simulink model "ODE_Hand_Model_v08_IPC_v02"  (Simulink 7.5)
settings: Solver=FixedStepDiscrete  StartTime=0.0  StopTime=inf  FixedStep=0.0315/(4*12)  RelTol=1e-3
values from neighbouring files (symbols this model uses):
  f_step = 0.7    [Set_Parameters.m]
  force_step = 20    [Set_Parameters.m]
  K_Conn = eye(4)*k_conn    [Set_Parameters.m]
  K_D = 30    [Set_Parameters.m]
  K_Or = eye(3)*k_Or    [Set_Parameters.m]
  K_Ot = eye(3)*k_Ot    [Set_Parameters.m]
  K_P = 350    [Set_Parameters.m]
  ksi = 2.0    (= 2)    [Set_Parameters.m]
  Kx = diag([diag(K_Ot)' diag(K_Or)' diag(K_Conn)'])    [Set_Parameters.m]
  l_des = [l1_des; l2_des; l3_des; l4_des]    [Set_Parameters.m]
  Mo = diag([sphere_mass*ones(1,3) (2/5)*sphere_mass*sphere_radius^2*ones(1,3)])    [Set_Parameters.m]
  qd_initial_touch = [0 0.3655   -0.5897   -0.5897     0       -0.3333   +0.5942   +0.5942         0       -0.298   --0.5226   --0.5226           0       -0.3333   +0.5942   +0.5942]    [Set_Parameters.m]
  R_O_Desired = R_O(x_i(qd_initial_touch))    [Set_Parameters.m]
  t_f_start = 2.5    [Set_Parameters.m]
  torque_step = 60    [Set_Parameters.m]
  x_O_desired = (1/4)*sum(x_i(qd_initial_touch))    [Set_Parameters.m]
undefined symbols (not defined in the file or in its folder): sigbuilder_block, skew
libraries: dspmtrx3 x29, simulink x4, dspinverses x1
settings Model: Creator=nihil  LastModifiedBy=konstantinos  SimulationMode=external
settings HardwareCC: ProdIntDivRoundTo=Zero  ProdEndianess=LittleEndian  ProdHWDeviceType=Generic->32-bit x86 compatible
settings RTWCC: SystemTargetFile=rtwin.tlc  TemplateMakefile=rtwin.tmf  Description=Real-Time Windows Target  ProcessScript=rtwin_make_rtw_hook  RTWCompilerOptimization=On
settings CodeAppCC: MaxIdLength=95
settings RTWinTargetCC: TargetLibSuffix=_rtwin.lib  TargetPreCompLibLocation=C:\Program Files (x86)\MATLAB\R2010a\toolbox\rtw\targets\rtwin\lib  TargetFunctionLibrary=ANSI_C  ERTCodeCoverageTool=None  PortableWordSizes=off

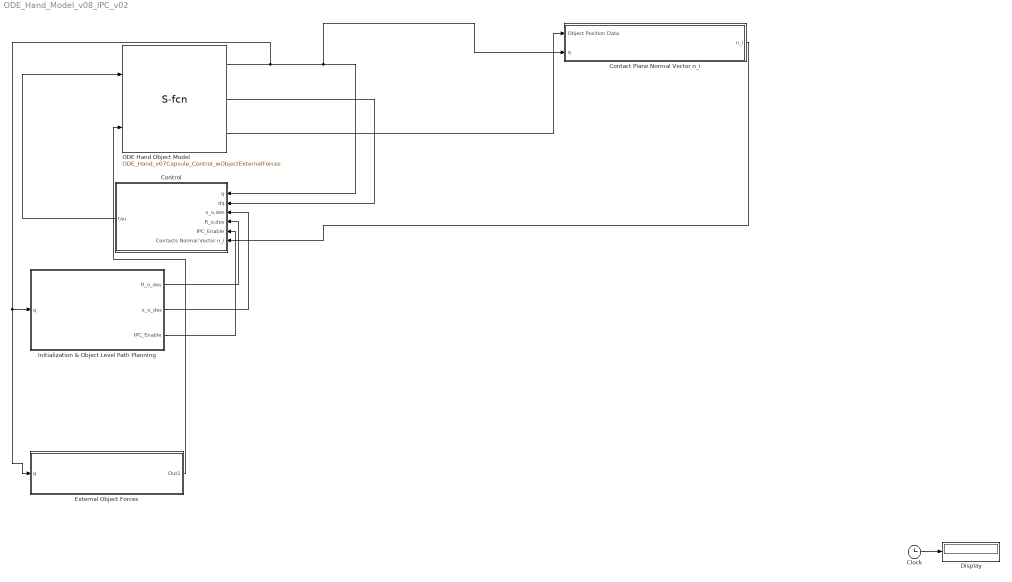
== system ODE_Hand_Model_v08_IPC_v02 ==
  Clock : Clock
      settings: Decimation=10
  Contact Plane Normal Vector n_i : Subsystem
  Control : Subsystem
  Display : Display
  External Object Forces : Subsystem
  Initialization & Object Level Path Planning : Subsystem
  ODE Hand Object Model : S-Function  FunctionName=ODE_Hand_v07Capsule_Control_wObjectExternalForces  EnableBusSupport=off
  wires:
  Clock/1 -> Display/1
  Control/1(tau) -> ODE Hand Object Model/1
  ODE Hand Object Model/1 -> Contact Plane Normal Vector n_i/2(q), Control/1(q), External Object Forces/1(q), Initialization & Object Level Path Planning/1(q)
  ODE Hand Object Model/2 -> Control/2(dq)
  Initialization & Object Level Path Planning/2(x_o_des) -> Control/3(x_o,des)
  Initialization & Object Level Path Planning/1(R_o_des) -> Control/4(R_o,des)
  Initialization & Object Level Path Planning/3(IPC_Enable) -> Control/5(IPC_Enable)
  External Object Forces/1(Out1) -> ODE Hand Object Model/2
  Contact Plane Normal Vector n_i/1(n_i) -> Control/6(Contacts Normal Vector n_i)
  ODE Hand Object Model/3 -> Contact Plane Normal Vector n_i/1(Object Position Data)

== system ODE_Hand_Model_v08_IPC_v02/Contact Plane Normal Vector n_i ==
  Object Position Data : Inport  OutDataType=fixdt(1, 16)  OutScaling=2^0
  q : Inport  Port=2  OutDataType=fixdt(1, 16)  OutScaling=2^0
  Cylindrical Object : Subsystem
  Manual Switch : simulink/Signal Routing/Manual Switch  SystemSampleTime=-1  sw=0  action=0  varsize=off
  Sphere : Subsystem
  x_i : MATLABFcn  MATLABFcn=x_i  Output1D=off
  n_i : Outport  OutDataType=fixdt(1, 16)  OutScaling=2^0
  wires:
  Object Position Data/1 -> Sphere/1(In1), Cylindrical Object/1(Position_Orientation)
  Sphere/1(Out1) -> Manual Switch/1
  Cylindrical Object/1(Out1) -> Manual Switch/2
  Manual Switch/1 -> n_i/1
  x_i/1 -> Cylindrical Object/2(x_i), Sphere/2(In2)
  q/1 -> x_i/1

== system ODE_Hand_Model_v08_IPC_v02/Control ==
  q : Inport  OutDataType=fixdt(1, 16)  OutScaling=2^0
  dq : Inport  Port=2  OutDataType=fixdt(1, 16)  OutScaling=2^0
  x_o,des : Inport  Port=3  OutDataType=fixdt(1, 16)  OutScaling=2^0
  R_o,des : Inport  Port=4  OutDataType=fixdt(1, 16)  OutScaling=2^0
  IPC_Enable : Inport  Port=5  OutDataType=fixdt(1, 16)  OutScaling=2^0
  Contacts Normal Vector n_i : Inport  Port=6  OutDataType=fixdt(1, 16)  OutScaling=2^0
  IPC : Subsystem
  Initial_Posture : Subsystem
  Switch : Switch  OutDataType=fixdt(1, 16)  OutScaling=2^0
  tau : Outport  OutDataType=fixdt(1, 16)  OutScaling=2^0
  wires:
  q/1 -> IPC/1(q), Initial_Posture/1(q)
  dq/1 -> IPC/2(dq), Initial_Posture/2(dq)
  Switch/1 -> tau/1
  Initial_Posture/1(Out1) -> Switch/3
  x_o,des/1 -> IPC/3(x_o,des)
  R_o,des/1 -> IPC/4(R_o,des)
  IPC/1(tau) -> Switch/1
  IPC_Enable/1 -> Switch/2
  Contacts Normal Vector n_i/1 -> IPC/5(n_i)

== system ODE_Hand_Model_v08_IPC_v02/External Object Forces ==
  q : Inport  OutDataType=fixdt(1, 16)  OutScaling=2^0
  Apply Force : Subsystem
  Apply Torque : Subsystem
  Display : Display
  Force--Torque : simulink/Signal Routing/Manual Switch  SystemSampleTime=-1  sw=1  action=0  varsize=off
  Gain : Gain  Gain=0  ParameterDataType=fixdt(1, 16)  ParameterScaling=2^0  OutDataType=fixdt(1, 16)  OutScaling=2^0
  Mux1 : Mux
  Mux2 : Mux  Inputs=3
  Mux3 : Mux
  Object Gravity OFF1 : Constant  OutDataType=fixdt(1, 16)  OutScaling=2^0
  Object Gravity ON : Constant  Value=0  OutDataType=fixdt(1, 16)  OutScaling=2^0
  Object_Gravity OFF-ON : simulink/Signal Routing/Manual Switch  SystemSampleTime=-1  sw=1  action=0  varsize=off
  Zero_the Rest : Constant  Value=zeros(1,16-13)  OutDataType=fixdt(1, 16)  OutScaling=2^0
  Out1 : Outport  OutDataType=fixdt(1, 16)  OutScaling=2^0
  wires:
  Object Gravity OFF1/1 -> Object_Gravity OFF-ON/1
  Object Gravity ON/1 -> Object_Gravity OFF-ON/2
  Mux2/1 -> Out1/1, Display/1
  q/1 -> Apply Force/1(In1), Apply Torque/1(In1)
  Zero_the Rest/1 -> Mux2/3
  Object_Gravity OFF-ON/1 -> Mux2/2
  Mux1/1 -> Force--Torque/1
  Mux3/1 -> Force--Torque/2
  Apply Force/1(Out1) -> Mux1/1
  Apply Force/2(Out2) -> Mux1/2
  Apply Force/3(Out3) -> Mux1/3
  Apply Force/4(Out4) -> Mux1/4
  Apply Torque/1(Out1) -> Mux3/1
  Apply Torque/2(Out2) -> Mux3/2
  Apply Torque/3(Out3) -> Mux3/3
  Apply Torque/4(Out4) -> Mux3/4
  Force--Torque/1 -> Gain/1
  Gain/1 -> Mux2/1

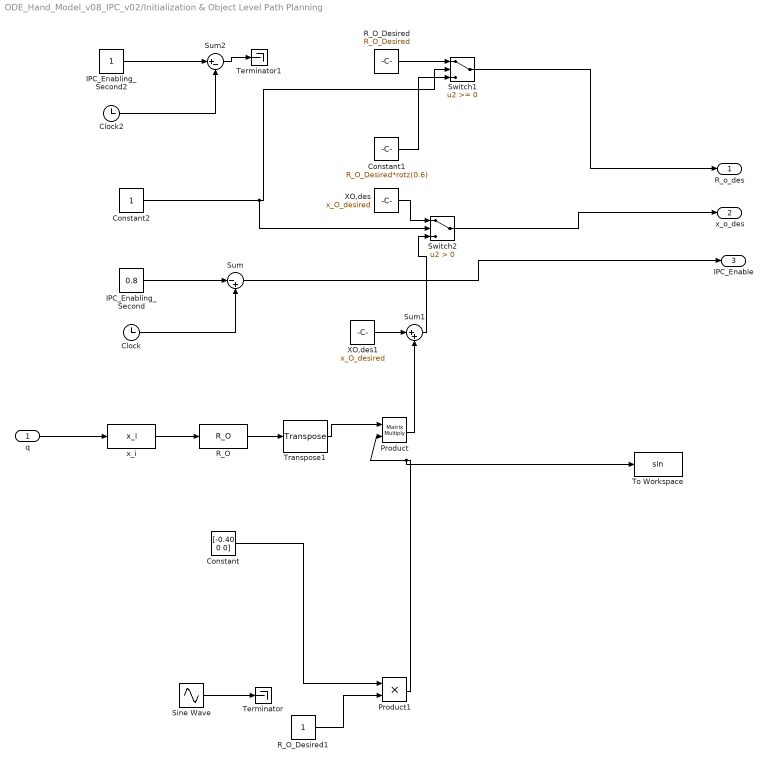
== system ODE_Hand_Model_v08_IPC_v02/Initialization & Object Level Path Planning ==
  q : Inport  OutDataType=fixdt(1, 16)  OutScaling=2^0
  Clock : Clock
      settings: Decimation=10
  Clock2 : Clock
      settings: Decimation=10
  Constant : Constant  Value=[-0.40 0 0]  OutDataType=fixdt(1, 16)  OutScaling=2^0
  Constant1 : Constant  Value=R_O_Desired*rotz(0.6)  OutDataType=fixdt(1, 16)  OutScaling=2^0
  Constant2 : Constant  OutDataType=fixdt(1, 16)  OutScaling=2^0
  IPC_Enabling_Second : Constant  Value=0.8  OutDataType=fixdt(1, 16)  OutScaling=2^0
  IPC_Enabling_Second2 : Constant  OutDataType=fixdt(1, 16)  OutScaling=2^0
  Product : Product  Multiplication=Matrix(*)  OutDataType=fixdt(1, 16)  OutScaling=2^0  RndMeth=Zero
  Product1 : Product  OutDataType=fixdt(1, 16)  OutScaling=2^0  RndMeth=Zero
  R_O : MATLABFcn  MATLABFcn=R_O  OutputSignalType=real  Output1D=off
  R_O_Desired : Constant  Value=R_O_Desired  OutDataType=fixdt(1, 16)  OutScaling=2^0
  R_O_Desired1 : Constant  OutDataType=fixdt(1, 16)  OutScaling=2^0
  Sine Wave : Sin  Amplitude=0.7  Bias=0  Frequency=4  Phase=0  Samples=10  SampleTime=0  Offset=0
  Sum : Sum  Inputs=|-+  OutDataType=fixdt(1, 16)  OutScaling=2^0
  Sum1 : Sum  Inputs=|++  OutDataType=fixdt(1, 16)  OutScaling=2^0
  Sum2 : Sum  Inputs=|+-  OutDataType=fixdt(1, 16)  OutScaling=2^0
  Switch1 : Switch  OutDataType=fixdt(1, 16)  OutScaling=2^0
  Switch2 : Switch  Criteria=u2 > Threshold  OutDataType=fixdt(1, 16)  OutScaling=2^0
  Terminator : Terminator
  Terminator1 : Terminator
  To Workspace : ToWorkspace  VariableName=sin  SampleTime=-1  SaveFormat=Structure
  Transpose1 : dspmtrx3/Transpose  SystemSampleTime=-1  Hermitian=off  overflowFlag=off
  XO,des : Constant  Value=x_O_desired  OutDataType=fixdt(1, 16)  OutScaling=2^0
  XO,des1 : Constant  Value=x_O_desired  OutDataType=fixdt(1, 16)  OutScaling=2^0
  x_i : MATLABFcn  MATLABFcn=x_i  Output1D=off
  R_o_des : Outport  OutDataType=fixdt(1, 16)  OutScaling=2^0
  x_o_des : Outport  Port=2  OutDataType=fixdt(1, 16)  OutScaling=2^0
  IPC_Enable : Outport  Port=3  OutDataType=fixdt(1, 16)  OutScaling=2^0
  wires:
  Clock/1 -> Sum/2
  IPC_Enabling_Second/1 -> Sum/1
  Sum/1 -> IPC_Enable/1
  R_O_Desired/1 -> Switch1/1
  Switch1/1 -> R_o_des/1
  Switch2/1 -> x_o_des/1
  Constant1/1 -> Switch1/3
  Clock2/1 -> Sum2/2
  IPC_Enabling_Second2/1 -> Sum2/1
  q/1 -> x_i/1
  x_i/1 -> R_O/1
  R_O/1 -> Transpose1/1
  Transpose1/1 -> Product/1
  XO,des1/1 -> Sum1/1
  Product/1 -> Sum1/2
  Sum1/1 -> Switch2/3
  Constant2/1 -> Switch1/2, Switch2/2
  XO,des/1 -> Switch2/1
  Constant/1 -> Product1/1
  Product1/1 -> Product/2, To Workspace/1
  Sine Wave/1 -> Terminator/1
  R_O_Desired1/1 -> Product1/2
  Sum2/1 -> Terminator1/1

== system ODE_Hand_Model_v08_IPC_v02/Contact Plane Normal Vector n_i/Cylindrical Object ==
  Position_Orientation : Inport  OutDataType=fixdt(1, 16)  OutScaling=2^0
  x_i : Inport  Port=2  OutDataType=fixdt(1, 16)  OutScaling=2^0
  MATLAB Fcn1 : MATLABFcn  MATLABFcn=[u(1,:) u(2,:) u(3,:) u(4,:)]
  Mux : Mux  Inputs=3
  Position : MATLABFcn  MATLABFcn=[u(1:3)]
  Position1 : MATLABFcn  MATLABFcn=Cylinder_n_i
  orientation : MATLABFcn  MATLABFcn=[u(4:6)]
  Out1 : Outport  OutDataType=fixdt(1, 16)  OutScaling=2^0
  wires:
  x_i/1 -> MATLAB Fcn1/1
  Position_Orientation/1 -> Position/1, orientation/1
  Position/1 -> Mux/1
  orientation/1 -> Mux/2
  MATLAB Fcn1/1 -> Mux/3
  Mux/1 -> Position1/1
  Position1/1 -> Out1/1

== system ODE_Hand_Model_v08_IPC_v02/Contact Plane Normal Vector n_i/Sphere ==
  In1 : Inport  OutDataType=fixdt(1, 16)  OutScaling=2^0
  In2 : Inport  Port=2  OutDataType=fixdt(1, 16)  OutScaling=2^0
  MATLAB Fcn : MATLABFcn  MATLABFcn=Sphere_n_i
  MATLAB Fcn1 : MATLABFcn  MATLABFcn=[u(1,:) u(2,:) u(3,:) u(4,:)]
  MATLAB Fcn2 : MATLABFcn  MATLABFcn=[u(1:3)]
  Mux : Mux  Inputs=2
  Out1 : Outport  OutDataType=fixdt(1, 16)  OutScaling=2^0
  wires:
  MATLAB Fcn/1 -> Out1/1
  In2/1 -> MATLAB Fcn1/1
  MATLAB Fcn1/1 -> Mux/2
  Mux/1 -> MATLAB Fcn/1
  In1/1 -> MATLAB Fcn2/1
  MATLAB Fcn2/1 -> Mux/1

== system ODE_Hand_Model_v08_IPC_v02/Control/IPC ==
  q : Inport  OutDataType=fixdt(1, 16)  OutScaling=2^0
  dq : Inport  Port=2  OutDataType=fixdt(1, 16)  OutScaling=2^0
  x_o,des : Inport  Port=3  OutDataType=fixdt(1, 16)  OutScaling=2^0
  R_o,des : Inport  Port=4  OutDataType=fixdt(1, 16)  OutScaling=2^0
  n_i : Inport  Port=5  OutDataType=fixdt(1, 16)  OutScaling=2^0
  Finger Gravity Compensation : MATLABFcn  MATLABFcn=gravity_dynamic_term  Output1D=off
  Finger Redundancy Controller : Subsystem
  J : Subsystem
  Object Level Damping(theta) : Subsystem
  "Object Level Stiffnes " : Subsystem
  Sum : Sum  Inputs=|---+  OutDataType=fixdt(1, 16)  OutScaling=2^0
  tau : Outport  OutDataType=fixdt(1, 16)  OutScaling=2^0
  wires:
  q/1 -> Finger Gravity Compensation/1, Object Level Damping(theta)/1(q), J/1(q), "Object Level Stiffnes "/1(q), Finger Redundancy Controller/1(q)
  Sum/1 -> tau/1
  dq/1 -> Object Level Damping(theta)/3(dq), Finger Redundancy Controller/2(dq)
  "Object Level Stiffnes "/1(Out1) -> Sum/2
  Object Level Damping(theta)/1(Out1) -> Sum/3
  J/1(J_Ot) -> "Object Level Stiffnes "/2(J_Ot)
  J/2(J_Or) -> "Object Level Stiffnes "/3(J_Or)
  J/4(J_tot) -> Object Level Damping(theta)/2(J_tot)
  Finger Gravity Compensation/1 -> Sum/4
  Finger Redundancy Controller/1(tau) -> Sum/1
  x_o,des/1 -> J/2(x_o,des), "Object Level Stiffnes "/5(x_o,des)
  J/3(JConn) -> "Object Level Stiffnes "/4(JConn)
  R_o,des/1 -> "Object Level Stiffnes "/6(R_o,des)
  J/5(J_H) -> "Object Level Stiffnes "/7(J_H)
  n_i/1 -> "Object Level Stiffnes "/8(n_i)

== system ODE_Hand_Model_v08_IPC_v02/Control/Initial_Posture ==
  q : Inport  OutDataType=fixdt(1, 16)  OutScaling=2^0
  dq : Inport  Port=2  OutDataType=fixdt(1, 16)  OutScaling=2^0
  Gain : Gain  Gain=K_P  ParameterDataType=fixdt(1, 16)  ParameterScaling=2^0  OutDataType=fixdt(1, 16)  OutScaling=2^0
  Gain1 : Gain  Gain=K_D  ParameterDataType=fixdt(1, 16)  ParameterScaling=2^0  OutDataType=fixdt(1, 16)  OutScaling=2^0
  Gravity Compensation : MATLABFcn  MATLABFcn=gravity_dynamic_term
  Ramp_Singals_qd : Subsystem
  Sum : Sum  Inputs=|--+  OutDataType=fixdt(1, 16)  OutScaling=2^0
  Sum1 : Sum  Inputs=|-+  OutDataType=fixdt(1, 16)  OutScaling=2^0
  Out1 : Outport  OutDataType=fixdt(1, 16)  OutScaling=2^0
  wires:
  q/1 -> Gravity Compensation/1, Sum1/2
  Sum/1 -> Out1/1
  Sum1/1 -> Gain/1
  dq/1 -> Gain1/1
  Gain1/1 -> Sum/1
  Gain/1 -> Sum/2
  Gravity Compensation/1 -> Sum/3
  Ramp_Singals_qd/1(Out1) -> Sum1/1

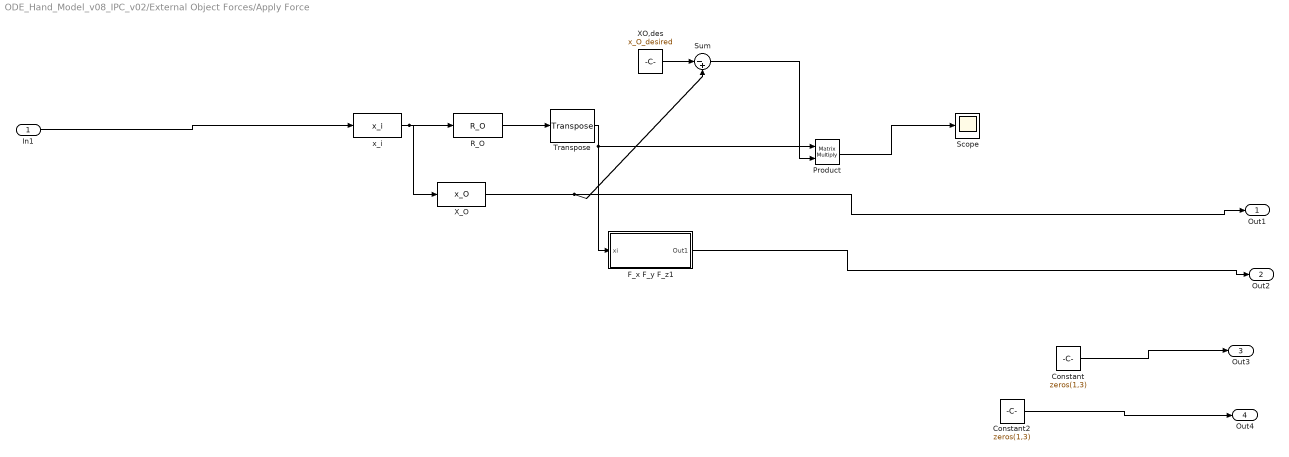
== system ODE_Hand_Model_v08_IPC_v02/External Object Forces/Apply Force ==
  In1 : Inport  OutDataType=fixdt(1, 16)  OutScaling=2^0
  Constant : Constant  Value=zeros(1,3)  VectorParams1D=off  OutDataType=fixdt(1, 16)  OutScaling=2^0
  Constant2 : Constant  Value=zeros(1,3)  VectorParams1D=off  OutDataType=fixdt(1, 16)  OutScaling=2^0
  F_x F_y F_z1 : Subsystem
  Product : Product  Multiplication=Matrix(*)  OutDataType=fixdt(1, 16)  OutScaling=2^0  RndMeth=Zero
  R_O : MATLABFcn  MATLABFcn=R_O  OutputSignalType=real  Output1D=off
  Scope : Scope
      settings: TimeRange=10  YMin=-0.45  YMax=0.075  SaveName=x_o
  Sum : Sum  Inputs=|-+  OutDataType=fixdt(1, 16)  OutScaling=2^0
  Transpose : dspmtrx3/Transpose  SystemSampleTime=-1  Hermitian=off  overflowFlag=off
  XO,des : Constant  Value=x_O_desired  OutDataType=fixdt(1, 16)  OutScaling=2^0
  X_O : MATLABFcn  MATLABFcn=x_O
  x_i : MATLABFcn  MATLABFcn=x_i  Output1D=off
  Out1 : Outport  OutDataType=fixdt(1, 16)  OutScaling=2^0
  Out2 : Outport  Port=2  OutDataType=fixdt(1, 16)  OutScaling=2^0
  Out3 : Outport  Port=3  OutDataType=fixdt(1, 16)  OutScaling=2^0
  Out4 : Outport  Port=4  OutDataType=fixdt(1, 16)  OutScaling=2^0
  wires:
  x_i/1 -> R_O/1, X_O/1
  F_x F_y F_z1/1(Out1) -> Out2/1
  X_O/1 -> Sum/2, Out1/1
  R_O/1 -> Transpose/1
  Transpose/1 -> F_x F_y F_z1/1(xi), Product/1
  In1/1 -> x_i/1
  Constant/1 -> Out3/1
  Constant2/1 -> Out4/1
  XO,des/1 -> Sum/1
  Sum/1 -> Product/2
  Product/1 -> Scope/1

== system ODE_Hand_Model_v08_IPC_v02/External Object Forces/Apply Torque ==
  In1 : Inport  OutDataType=fixdt(1, 16)  OutScaling=2^0
  Subsystem : Subsystem
  Subsystem2 : Subsystem
  Out1 : Outport  OutDataType=fixdt(1, 16)  OutScaling=2^0
  Out2 : Outport  Port=2  OutDataType=fixdt(1, 16)  OutScaling=2^0
  Out3 : Outport  Port=3  OutDataType=fixdt(1, 16)  OutScaling=2^0
  Out4 : Outport  Port=4  OutDataType=fixdt(1, 16)  OutScaling=2^0
  wires:
  Subsystem/1(Out1) -> Out1/1
  Subsystem/2(Out2) -> Out2/1
  Subsystem2/1(Out1) -> Out3/1
  Subsystem2/2(Out2) -> Out4/1
  In1/1 -> Subsystem/1(In1), Subsystem2/1(In1)

== system ODE_Hand_Model_v08_IPC_v02/Control/IPC/Finger Redundancy Controller ==
  q : Inport  OutDataType=fixdt(1, 16)  OutScaling=2^0
  dq : Inport  Port=2  OutDataType=fixdt(1, 16)  OutScaling=2^0
  MATLAB Fcn : MATLABFcn  MATLABFcn=redundancy_controller
  Terminator : Terminator
  tau : Outport  OutDataType=fixdt(1, 16)  OutScaling=2^0
  wires:
  MATLAB Fcn/1 -> tau/1
  q/1 -> MATLAB Fcn/1
  dq/1 -> Terminator/1

== system ODE_Hand_Model_v08_IPC_v02/Control/IPC/J ==
  q : Inport  OutDataType=fixdt(1, 16)  OutScaling=2^0
  x_o,des : Inport  Port=2  OutDataType=fixdt(1, 16)  OutScaling=2^0
  JH : MATLABFcn  MATLABFcn=J_H  Output1D=off
  J_Or1 : Subsystem
  J_Ot1 : Subsystem
  Jconn : Subsystem
  Matrix Concatenate : Concatenate  NumInputs=3  Mode=Multidimensional array  ConcatenateDimension=2
  Transpose{,1..3} (4 alike) : dspmtrx3/Transpose  SystemSampleTime=-1  Hermitian=off  overflowFlag=off
  J_Ot : Outport  OutDataType=fixdt(1, 16)  OutScaling=2^0
  J_Or : Outport  Port=2  OutDataType=fixdt(1, 16)  OutScaling=2^0
  JConn : Outport  Port=3  OutDataType=fixdt(1, 16)  OutScaling=2^0
  J_tot : Outport  Port=4  OutDataType=fixdt(1, 16)  OutScaling=2^0
  J_H : Outport  Port=5  OutDataType=fixdt(1, 16)  OutScaling=2^0
  wires:
  JH/1 -> Jconn/2(JH), J_Or1/2(J_H), J_Ot1/2(JH), J_H/1
  J_Or1/1(Out1) -> J_Ot1/3(J_Or), J_Or/1, Transpose1/1
  q/1 -> JH/1, Jconn/1(q), J_Or1/1(q), J_Ot1/1(q)
  J_Ot1/1(Out1) -> J_Ot/1, Transpose/1
  Jconn/1(Out1) -> JConn/1, Transpose2/1
  Transpose2/1 -> Matrix Concatenate/3
  Transpose1/1 -> Matrix Concatenate/2
  Transpose/1 -> Matrix Concatenate/1
  Matrix Concatenate/1 -> Transpose3/1
  Transpose3/1 -> J_tot/1
  x_o,des/1 -> J_Ot1/4(x_o,des)

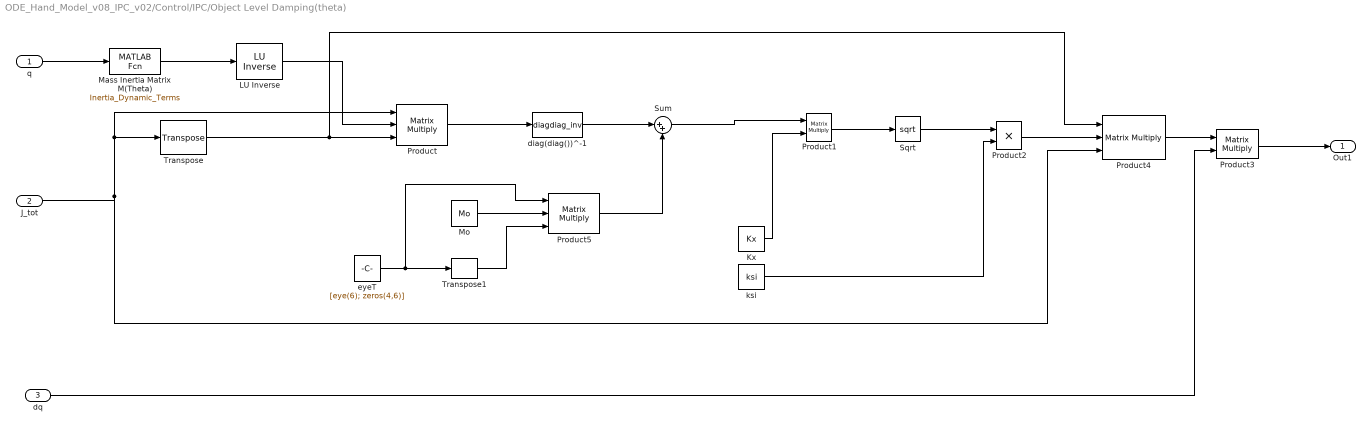
== system ODE_Hand_Model_v08_IPC_v02/Control/IPC/Object Level Damping(theta) ==
  q : Inport  OutDataType=fixdt(1, 16)  OutScaling=2^0
  J_tot : Inport  Port=2  OutDataType=fixdt(1, 16)  OutScaling=2^0
  dq : Inport  Port=3  OutDataType=fixdt(1, 16)  OutScaling=2^0
  " LU Inverse" : dspinverses/ LU Inverse  SystemSampleTime=-1
  Kx : Constant  Value=Kx  OutDataType=fixdt(1, 16)  OutScaling=2^0
  Mass Inertia Matrix M(Theta) : MATLABFcn  MATLABFcn=Inertia_Dynamic_Terms  Output1D=off
  Mo : Constant  Value=Mo  OutDataType=fixdt(1, 16)  OutScaling=2^0
  Product : Product  Inputs=3  Multiplication=Matrix(*)  OutDataType=fixdt(1, 16)  OutScaling=2^0  RndMeth=Zero
  Product1 : Product  Multiplication=Matrix(*)  OutDataType=fixdt(1, 16)  OutScaling=2^0  RndMeth=Zero
  Product2 : Product  OutDataType=fixdt(1, 16)  OutScaling=2^0  RndMeth=Zero
  Product3 : Product  Multiplication=Matrix(*)  OutDataType=fixdt(1, 16)  OutScaling=2^0  RndMeth=Zero
  Product4 : Product  Inputs=3  Multiplication=Matrix(*)  OutDataType=fixdt(1, 16)  OutScaling=2^0  RndMeth=Zero
  Product5 : Product  Inputs=3  Multiplication=Matrix(*)  OutDataType=fixdt(1, 16)  OutScaling=2^0  RndMeth=Zero
  Sqrt : Sqrt  OutputSignalType=real  SaturateOnIntegerOverflow=on
  Sum : Sum  Inputs=|++  OutDataType=fixdt(1, 16)  OutScaling=2^0
  Transpose : dspmtrx3/Transpose  SystemSampleTime=-1  Hermitian=off  overflowFlag=off
  Transpose1 : dspmtrx3/Transpose  SystemSampleTime=-1  Hermitian=off  overflowFlag=off
  diag(diag())^-1 : MATLABFcn  MATLABFcn=diagdiag_inv  Output1D=off
  eyeT : Constant  Value=[eye(6); zeros(4,6)]  OutDataType=fixdt(1, 16)  OutScaling=2^0
  ksi : Constant  Value=ksi  OutDataType=fixdt(1, 16)  OutScaling=2^0
  Out1 : Outport  OutDataType=fixdt(1, 16)  OutScaling=2^0
  wires:
  q/1 -> Mass Inertia Matrix M(Theta)/1
  J_tot/1 -> Transpose/1, Product/1, Product4/3
  Transpose/1 -> Product/3, Product4/1
  Mass Inertia Matrix M(Theta)/1 -> " LU Inverse"/1
  " LU Inverse"/1 -> Product/2
  Product/1 -> diag(diag())^-1/1
  Sqrt/1 -> Product2/1
  ksi/1 -> Product2/2
  Product2/1 -> Product4/2
  Product4/1 -> Product3/1
  dq/1 -> Product3/2
  Product3/1 -> Out1/1
  Kx/1 -> Product1/2
  Product1/1 -> Sqrt/1
  eyeT/1 -> Transpose1/1, Product5/1
  Sum/1 -> Product1/1
  diag(diag())^-1/1 -> Sum/1
  Mo/1 -> Product5/2
  Transpose1/1 -> Product5/3
  Product5/1 -> Sum/2

== system ODE_Hand_Model_v08_IPC_v02/Control/IPC/Object Level Stiffnes  ==
  q : Inport  OutDataType=fixdt(1, 16)  OutScaling=2^0
  J_Ot : Inport  Port=2  OutDataType=fixdt(1, 16)  OutScaling=2^0
  J_Or : Inport  Port=3  OutDataType=fixdt(1, 16)  OutScaling=2^0
  JConn : Inport  Port=4  OutDataType=fixdt(1, 16)  OutScaling=2^0
  x_o,des : Inport  Port=5  OutDataType=fixdt(1, 16)  OutScaling=2^0
  R_o,des : Inport  Port=6  OutDataType=fixdt(1, 16)  OutScaling=2^0
  J_H : Inport  Port=7  OutDataType=fixdt(1, 16)  OutScaling=2^0
  n_i : Inport  Port=8  OutDataType=fixdt(1, 16)  OutScaling=2^0
  Manual Switch : simulink/Signal Routing/Manual Switch  SystemSampleTime=-1  sw=1  action=0  varsize=off
  Subsystem : Subsystem
  Sum : Sum  Inputs=|+++  OutDataType=fixdt(1, 16)  OutScaling=2^0
  VConn(theta) : Subsystem
  VO,r(theta) : Subsystem
  VO,t(theta) : Subsystem
  Out1 : Outport  OutDataType=fixdt(1, 16)  OutScaling=2^0
  wires:
  q/1 -> VConn(theta)/1(q), VO,r(theta)/1(q), VO,t(theta)/1(q), Subsystem/3(q)
  VO,r(theta)/1(Partial V_r) -> Sum/1
  Sum/1 -> Out1/1
  VO,t(theta)/1(Out1) -> Sum/2
  JConn/1 -> VConn(theta)/2(J_Conn)
  J_Ot/1 -> VO,t(theta)/2(JOt)
  J_Or/1 -> VO,r(theta)/2(JOr)
  x_o,des/1 -> VO,t(theta)/3(x_o,des)
  R_o,des/1 -> VO,r(theta)/3(R_o,des)
  VConn(theta)/1(Out1) -> Manual Switch/1
  Manual Switch/1 -> Sum/3
  J_H/1 -> Subsystem/1(J_H)
  n_i/1 -> Subsystem/2(n_i)
  Subsystem/1(Out1) -> Manual Switch/2

== system ODE_Hand_Model_v08_IPC_v02/Control/Initial_Posture/Ramp_Singals_qd ==
  Product : Product  OutDataType=fixdt(1, 16)  OutScaling=2^0  RndMeth=Zero
  Ramp : Subsystem  Tag=STV Subsys  LoadFcn=sigbuilder_block('load');  StartFcn=sigbuilder_block('start');  StopFcn=sigbuilder_block('stop');  ClipboardFcn=sigbuilder_block('clipboard');  mask(Sigbuilder block){}
      mask help: Create and generate interchangeable groups of signals whose waveforms are piecewise linear.
      mask init:
      | if ~strcmp(get_param(bdroot(gcbh),'SimulationStatus'),'stopped') tuvar = sigbuilder_block('maskInit'); end
      settings: CopyFcn=sigbuilder_block('copy');  DeleteFcn=sigbuilder_block('delete');  ModelCloseFcn=sigbuilder_block('modelClose');  PreSaveFcn=sigbuilder_block('preSave');  NameChangeFcn=sigbuilder_block('namechange');  OpenFcn=sigbuilder_block('open',[-1260 6 1260 531 ]);  CloseFcn=sigbuilder_block('close');
      mask Display: plot(0,0,100,100,[10,10,40,40,10],[80,20,20,80,80],[40,10],[50,50], [40,27,10],[65,72,56],[40,25,25,10],[28,28,43,43]);
  qd_initial_touch : Constant  Value=qd_initial_touch  OutDataType=fixdt(1, 16)  OutScaling=2^0
  Out1 : Outport  OutDataType=fixdt(1, 16)  OutScaling=2^0
  wires:
  Ramp/1(Signal 1) -> Product/1
  qd_initial_touch/1 -> Product/2
  Product/1 -> Out1/1

== system ODE_Hand_Model_v08_IPC_v02/External Object Forces/Apply Force/F_x F_y F_z1 ==
  xi : Inport  OutDataType=fixdt(1, 16)  OutScaling=2^0
  Constant : Constant  Value=0  OutDataType=fixdt(1, 16)  OutScaling=2^0
  Constant1 : Constant  Value=0  OutDataType=fixdt(1, 16)  OutScaling=2^0
  Fx Force Multiplier : Subsystem
  Mux : Mux  Inputs=3
  Product : Product  Multiplication=Matrix(*)  OutDataType=fixdt(1, 16)  OutScaling=2^0  RndMeth=Zero
  Out1 : Outport  OutDataType=fixdt(1, 16)  OutScaling=2^0
  wires:
  Mux/1 -> Product/2
  Product/1 -> Out1/1
  xi/1 -> Product/1
  Constant1/1 -> Mux/1
  Constant/1 -> Mux/2
  Fx Force Multiplier/1(Out1) -> Mux/3

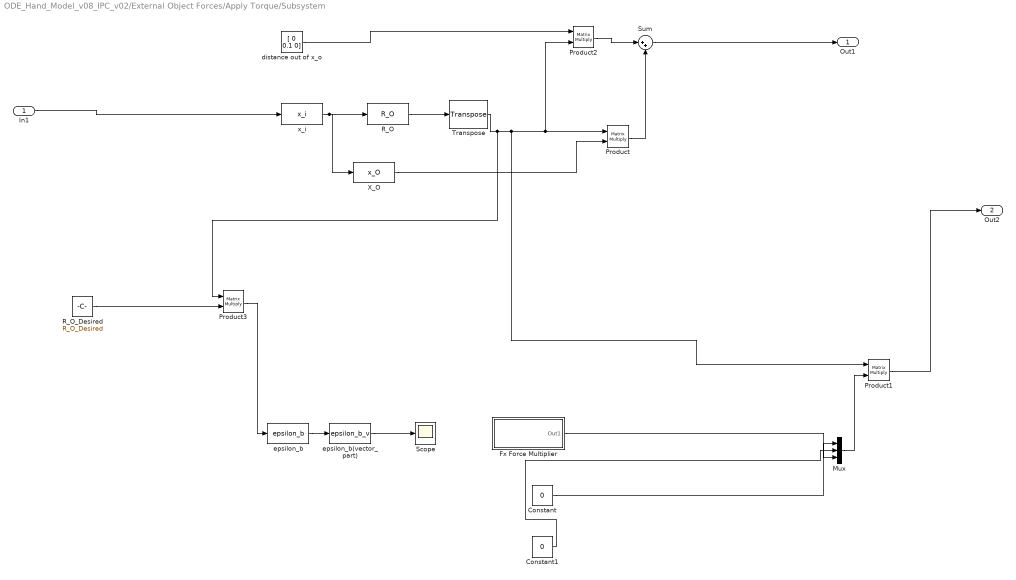
== system ODE_Hand_Model_v08_IPC_v02/External Object Forces/Apply Torque/Subsystem ==
  In1 : Inport  OutDataType=fixdt(1, 16)  OutScaling=2^0
  Constant : Constant  Value=0  OutDataType=fixdt(1, 16)  OutScaling=2^0
  Constant1 : Constant  Value=0  OutDataType=fixdt(1, 16)  OutScaling=2^0
  Fx Force Multiplier : Subsystem
  Mux : Mux  Inputs=3
  Product{,1..3} (4 alike) : Product  Multiplication=Matrix(*)  OutDataType=fixdt(1, 16)  OutScaling=2^0  RndMeth=Zero
  R_O : MATLABFcn  MATLABFcn=R_O  OutputSignalType=real  Output1D=off
  R_O_Desired : Constant  Value=R_O_Desired  OutDataType=fixdt(1, 16)  OutScaling=2^0
  Scope : Scope
      settings: YMin=-0.325  YMax=0.05  SaveName=e_b
  Sum : Sum  Inputs=|++  OutDataType=fixdt(1, 16)  OutScaling=2^0
  Transpose : dspmtrx3/Transpose  SystemSampleTime=-1  Hermitian=off  overflowFlag=off
  X_O : MATLABFcn  MATLABFcn=x_O
  distance out of x_o : Constant  Value="[  0 0.1 0]"  VectorParams1D=off  OutDataType=fixdt(1, 16)  OutScaling=2^0
  epsilon_b : MATLABFcn  MATLABFcn=epsilon_b  Output1D=off
  epsilon_b(vector_part) : MATLABFcn  MATLABFcn=epsilon_b_v  Output1D=off
  x_i : MATLABFcn  MATLABFcn=x_i  Output1D=off
  Out1 : Outport  OutDataType=fixdt(1, 16)  OutScaling=2^0
  Out2 : Outport  Port=2  OutDataType=fixdt(1, 16)  OutScaling=2^0
  wires:
  x_i/1 -> R_O/1, X_O/1
  X_O/1 -> Product/2
  R_O/1 -> Transpose/1
  Transpose/1 -> Product1/1, Product/1, Product2/2, Product3/1
  In1/1 -> x_i/1
  Product/1 -> Sum/2
  Mux/1 -> Product1/2
  distance out of x_o/1 -> Product2/1
  Product2/1 -> Sum/1
  Sum/1 -> Out1/1
  Product1/1 -> Out2/1
  Product3/1 -> epsilon_b/1
  epsilon_b/1 -> epsilon_b(vector_part)/1
  epsilon_b(vector_part)/1 -> Scope/1
  R_O_Desired/1 -> Product3/2
  Constant1/1 -> Mux/2
  Constant/1 -> Mux/1
  Fx Force Multiplier/1(Out1) -> Mux/3

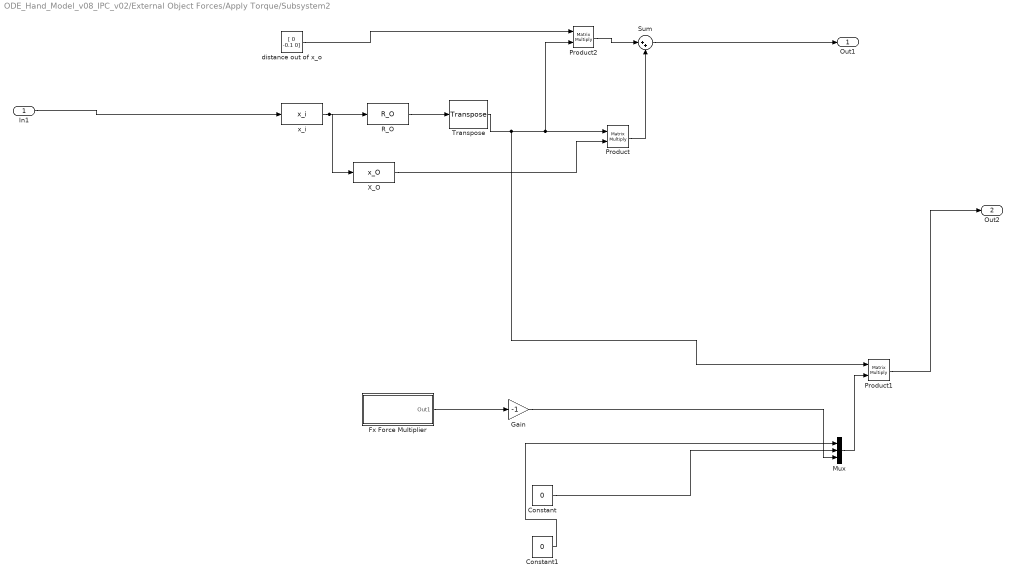
== system ODE_Hand_Model_v08_IPC_v02/External Object Forces/Apply Torque/Subsystem2 ==
  In1 : Inport  OutDataType=fixdt(1, 16)  OutScaling=2^0
  Constant : Constant  Value=0  OutDataType=fixdt(1, 16)  OutScaling=2^0
  Constant1 : Constant  Value=0  OutDataType=fixdt(1, 16)  OutScaling=2^0
  Fx Force Multiplier : Subsystem
  Gain : Gain  Gain=-1  ParameterDataType=fixdt(1, 16)  ParameterScaling=2^0  OutDataType=fixdt(1, 16)  OutScaling=2^0
  Mux : Mux  Inputs=3
  Product : Product  Multiplication=Matrix(*)  OutDataType=fixdt(1, 16)  OutScaling=2^0  RndMeth=Zero
  Product1 : Product  Multiplication=Matrix(*)  OutDataType=fixdt(1, 16)  OutScaling=2^0  RndMeth=Zero
  Product2 : Product  Multiplication=Matrix(*)  OutDataType=fixdt(1, 16)  OutScaling=2^0  RndMeth=Zero
  R_O : MATLABFcn  MATLABFcn=R_O  OutputSignalType=real  Output1D=off
  Sum : Sum  Inputs=|++  OutDataType=fixdt(1, 16)  OutScaling=2^0
  Transpose : dspmtrx3/Transpose  SystemSampleTime=-1  Hermitian=off  overflowFlag=off
  X_O : MATLABFcn  MATLABFcn=x_O
  distance out of x_o : Constant  Value="[ 0  -0.1 0]"  VectorParams1D=off  OutDataType=fixdt(1, 16)  OutScaling=2^0
  x_i : MATLABFcn  MATLABFcn=x_i  Output1D=off
  Out1 : Outport  OutDataType=fixdt(1, 16)  OutScaling=2^0
  Out2 : Outport  Port=2  OutDataType=fixdt(1, 16)  OutScaling=2^0
  wires:
  x_i/1 -> R_O/1, X_O/1
  X_O/1 -> Product/2
  R_O/1 -> Transpose/1
  Transpose/1 -> Product1/1, Product/1, Product2/2
  In1/1 -> x_i/1
  Product/1 -> Sum/2
  Mux/1 -> Product1/2
  distance out of x_o/1 -> Product2/1
  Product2/1 -> Sum/1
  Sum/1 -> Out1/1
  Product1/1 -> Out2/1
  Fx Force Multiplier/1(Out1) -> Gain/1
  Constant/1 -> Mux/2
  Constant1/1 -> Mux/1
  Gain/1 -> Mux/3

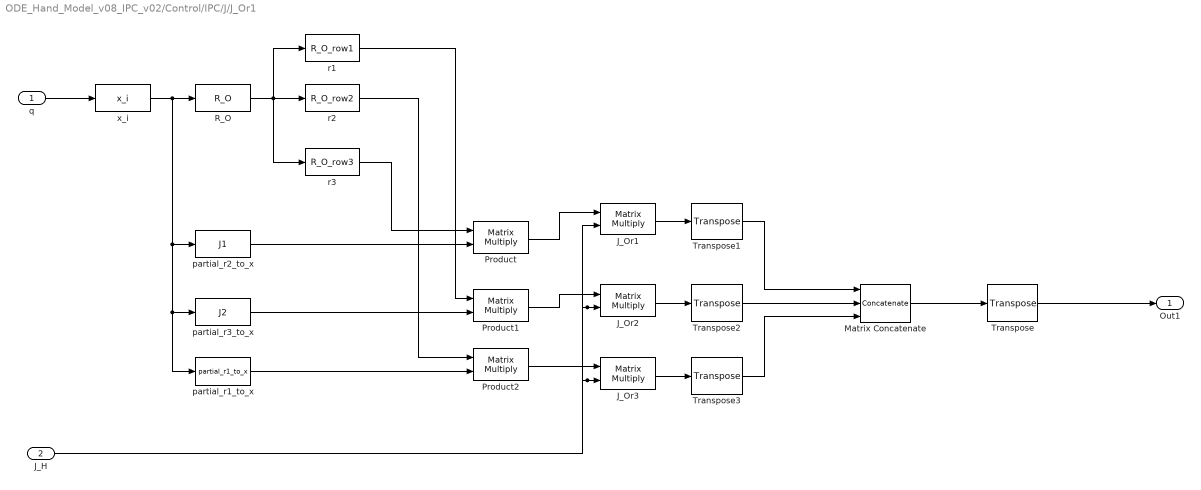
== system ODE_Hand_Model_v08_IPC_v02/Control/IPC/J/J_Or1 ==
  q : Inport  OutDataType=fixdt(1, 16)  OutScaling=2^0
  J_H : Inport  Port=2  OutDataType=fixdt(1, 16)  OutScaling=2^0
  J_Or1 : Product  Multiplication=Matrix(*)  OutDataType=fixdt(1, 16)  OutScaling=2^0  RndMeth=Zero
  J_Or2 : Product  Multiplication=Matrix(*)  OutDataType=fixdt(1, 16)  OutScaling=2^0  RndMeth=Zero
  J_Or3 : Product  Multiplication=Matrix(*)  OutDataType=fixdt(1, 16)  OutScaling=2^0  RndMeth=Zero
  Matrix Concatenate : Concatenate  NumInputs=3  Mode=Multidimensional array  ConcatenateDimension=2
  Product : Product  Multiplication=Matrix(*)  OutDataType=fixdt(1, 16)  OutScaling=2^0  RndMeth=Zero
  Product1 : Product  Multiplication=Matrix(*)  OutDataType=fixdt(1, 16)  OutScaling=2^0  RndMeth=Zero
  Product2 : Product  Multiplication=Matrix(*)  OutDataType=fixdt(1, 16)  OutScaling=2^0  RndMeth=Zero
  R_O : MATLABFcn  MATLABFcn=R_O  OutputSignalType=real  Output1D=off
  Transpose{,1..3} (4 alike) : dspmtrx3/Transpose  SystemSampleTime=-1  Hermitian=off  overflowFlag=off
  partial_r1_to_x : MATLABFcn  MATLABFcn=partial_r1_to_x  Output1D=off
  partial_r2_to_x : MATLABFcn  MATLABFcn=J1  Output1D=off
  partial_r3_to_x : MATLABFcn  MATLABFcn=J2  Output1D=off
  r1 : MATLABFcn  MATLABFcn=R_O_row1  OutputSignalType=real  Output1D=off
  r2 : MATLABFcn  MATLABFcn=R_O_row2  OutputSignalType=real  Output1D=off
  r3 : MATLABFcn  MATLABFcn=R_O_row3  OutputSignalType=real  Output1D=off
  x_i : MATLABFcn  MATLABFcn=x_i  Output1D=off
  Out1 : Outport  OutDataType=fixdt(1, 16)  OutScaling=2^0
  wires:
  x_i/1 -> partial_r2_to_x/1, partial_r3_to_x/1, partial_r1_to_x/1, R_O/1
  q/1 -> x_i/1
  Product/1 -> J_Or1/1
  Product1/1 -> J_Or2/1
  Product2/1 -> J_Or3/1
  J_H/1 -> J_Or2/2, J_Or1/2, J_Or3/2
  Matrix Concatenate/1 -> Transpose/1
  Transpose/1 -> Out1/1
  J_Or1/1 -> Transpose1/1
  J_Or2/1 -> Transpose2/1
  J_Or3/1 -> Transpose3/1
  Transpose2/1 -> Matrix Concatenate/2
  Transpose1/1 -> Matrix Concatenate/1
  Transpose3/1 -> Matrix Concatenate/3
  r1/1 -> Product1/1
  r2/1 -> Product2/1
  r3/1 -> Product/1
  partial_r2_to_x/1 -> Product/2
  partial_r3_to_x/1 -> Product1/2
  partial_r1_to_x/1 -> Product2/2
  R_O/1 -> r2/1, r1/1, r3/1

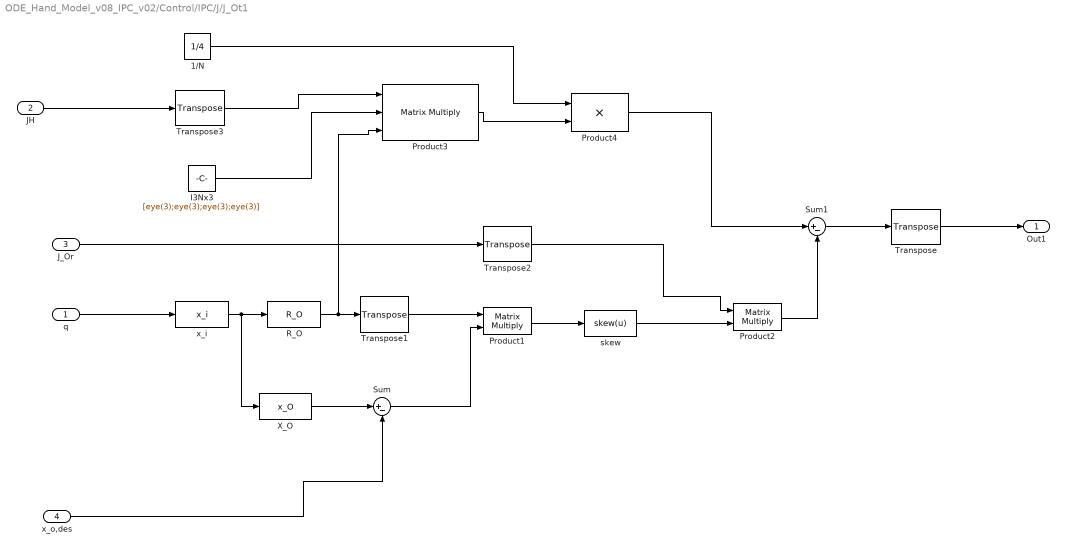
== system ODE_Hand_Model_v08_IPC_v02/Control/IPC/J/J_Ot1 ==
  q : Inport  OutDataType=fixdt(1, 16)  OutScaling=2^0
  JH : Inport  Port=2  OutDataType=fixdt(1, 16)  OutScaling=2^0
  J_Or : Inport  Port=3  OutDataType=fixdt(1, 16)  OutScaling=2^0
  x_o,des : Inport  Port=4  OutDataType=fixdt(1, 16)  OutScaling=2^0
  1/N : Constant  Value=1/4  OutDataType=fixdt(1, 16)  OutScaling=2^0
  I3Nx3 : Constant  Value=[eye(3);eye(3);eye(3);eye(3)]  OutDataType=fixdt(1, 16)  OutScaling=2^0
  Product1 : Product  Multiplication=Matrix(*)  OutDataType=fixdt(1, 16)  OutScaling=2^0  RndMeth=Zero
  Product2 : Product  Multiplication=Matrix(*)  OutDataType=fixdt(1, 16)  OutScaling=2^0  RndMeth=Zero
  Product3 : Product  Inputs=3  Multiplication=Matrix(*)  OutDataType=fixdt(1, 16)  OutScaling=2^0  RndMeth=Zero
  Product4 : Product  OutDataType=fixdt(1, 16)  OutScaling=2^0  RndMeth=Zero
  R_O : MATLABFcn  MATLABFcn=R_O  OutputSignalType=real  Output1D=off
  Sum : Sum  Inputs=|+-  OutDataType=fixdt(1, 16)  OutScaling=2^0
  Sum1 : Sum  Inputs=|+-  OutDataType=fixdt(1, 16)  OutScaling=2^0
  Transpose{,1..3} (4 alike) : dspmtrx3/Transpose  SystemSampleTime=-1  Hermitian=off  overflowFlag=off
  X_O : MATLABFcn  MATLABFcn=x_O
  skew : MATLABFcn  MATLABFcn=skew(u)  Output1D=off
  x_i : MATLABFcn  MATLABFcn=x_i  Output1D=off
  Out1 : Outport  OutDataType=fixdt(1, 16)  OutScaling=2^0
  wires:
  q/1 -> x_i/1
  x_i/1 -> R_O/1, X_O/1
  R_O/1 -> Transpose1/1, Product3/3
  X_O/1 -> Sum/1
  x_o,des/1 -> Sum/2
  Sum/1 -> Product1/2
  Transpose1/1 -> Product1/1
  Product1/1 -> skew/1
  skew/1 -> Product2/2
  J_Or/1 -> Transpose2/1
  Transpose2/1 -> Product2/1
  Product2/1 -> Sum1/2
  Sum1/1 -> Transpose/1
  Transpose/1 -> Out1/1
  JH/1 -> Transpose3/1
  Transpose3/1 -> Product3/1
  I3Nx3/1 -> Product3/2
  Product3/1 -> Product4/2
  Product4/1 -> Sum1/1
  1/N/1 -> Product4/1

== system ODE_Hand_Model_v08_IPC_v02/Control/IPC/J/Jconn ==
  q : Inport  OutDataType=fixdt(1, 16)  OutScaling=2^0
  JH : Inport  Port=2  OutDataType=fixdt(1, 16)  OutScaling=2^0
  Product2 : Product  Multiplication=Matrix(*)  OutDataType=fixdt(1, 16)  OutScaling=2^0  RndMeth=Zero
  Transpose : dspmtrx3/Transpose  SystemSampleTime=-1  Hermitian=off  overflowFlag=off
  Transpose1 : dspmtrx3/Transpose  SystemSampleTime=-1  Hermitian=off  overflowFlag=off
  partial_x : MATLABFcn  MATLABFcn=partial_x  OutputSignalType=real  Output1D=off
  x_i : MATLABFcn  MATLABFcn=x_i  Output1D=off
  Out1 : Outport  OutDataType=fixdt(1, 16)  OutScaling=2^0
  wires:
  x_i/1 -> partial_x/1
  Transpose/1 -> Product2/1
  partial_x/1 -> Product2/2
  JH/1 -> Transpose/1
  q/1 -> x_i/1
  Product2/1 -> Transpose1/1
  Transpose1/1 -> Out1/1

== system ODE_Hand_Model_v08_IPC_v02/Control/IPC/Object Level Stiffnes /Subsystem ==
  J_H : Inport  OutDataType=fixdt(1, 16)  OutScaling=2^0
  n_i : Inport  Port=2  OutDataType=fixdt(1, 16)  OutScaling=2^0
  q : Inport  Port=3  OutDataType=fixdt(1, 16)  OutScaling=2^0
  F_normal : Constant  Value=F_normal'  OutDataType=fixdt(1, 16)  OutScaling=2^0
  Null! : MATLABFcn  MATLABFcn=NullSpaceProjection  Output1D=off
  Product : Product  Multiplication=Matrix(*)  OutDataType=fixdt(1, 16)  OutScaling=2^0  RndMeth=Zero
  Product1 : Product  Inputs=3  Multiplication=Matrix(*)  OutDataType=fixdt(1, 16)  OutScaling=2^0  RndMeth=Zero
  Transpose : dspmtrx3/Transpose  SystemSampleTime=-1  Hermitian=off  overflowFlag=off
  gsn : MATLABFcn  MATLABFcn=gsn  Output1D=off
  n : MATLABFcn  MATLABFcn=n  Output1D=off
  r_i : MATLABFcn  MATLABFcn=r_i  Output1D=off
  x_i : MATLABFcn  MATLABFcn=x_i  Output1D=off
  Out1 : Outport  OutDataType=fixdt(1, 16)  OutScaling=2^0
  wires:
  Product/1 -> Out1/1
  J_H/1 -> Transpose/1
  q/1 -> x_i/1
  n_i/1 -> n/1
  x_i/1 -> r_i/1
  r_i/1 -> gsn/1
  Product1/1 -> Product/2
  n/1 -> Product1/2
  F_normal/1 -> Product1/3
  Null!/1 -> Product1/1
  gsn/1 -> Null!/1
  Transpose/1 -> Product/1

== system ODE_Hand_Model_v08_IPC_v02/Control/IPC/Object Level Stiffnes /VConn(theta) ==
  q : Inport  OutDataType=fixdt(1, 16)  OutScaling=2^0
  J_Conn : Inport  Port=2  OutDataType=fixdt(1, 16)  OutScaling=2^0
  Delta_x : MATLABFcn  MATLABFcn=Delta_x  Output1D=off
  K_Conn : Constant  Value=K_Conn  OutDataType=fixdt(1, 16)  OutScaling=2^0
  Product : Product  Multiplication=Matrix(*)  OutDataType=fixdt(1, 16)  OutScaling=2^0  RndMeth=Zero
  Product1 : Product  Multiplication=Matrix(*)  OutDataType=fixdt(1, 16)  OutScaling=2^0  RndMeth=Zero
  Sum : Sum  Inputs=|+-  OutDataType=fixdt(1, 16)  OutScaling=2^0
  Transpose : dspmtrx3/Transpose  SystemSampleTime=-1  Hermitian=off  overflowFlag=off
  Transpose1 : dspmtrx3/Transpose  SystemSampleTime=-1  Hermitian=off  overflowFlag=off
  l_des : Constant  Value=l_des  OutDataType=fixdt(1, 16)  OutScaling=2^0
  x_i : MATLABFcn  MATLABFcn=x_i  Output1D=off
  Out1 : Outport  OutDataType=fixdt(1, 16)  OutScaling=2^0
  wires:
  q/1 -> x_i/1
  x_i/1 -> Delta_x/1
  Delta_x/1 -> Sum/1
  l_des/1 -> Sum/2
  Sum/1 -> Product/2
  Product/1 -> Product1/2
  K_Conn/1 -> Product/1
  J_Conn/1 -> Transpose/1
  Transpose/1 -> Product1/1
  Product1/1 -> Transpose1/1
  Transpose1/1 -> Out1/1

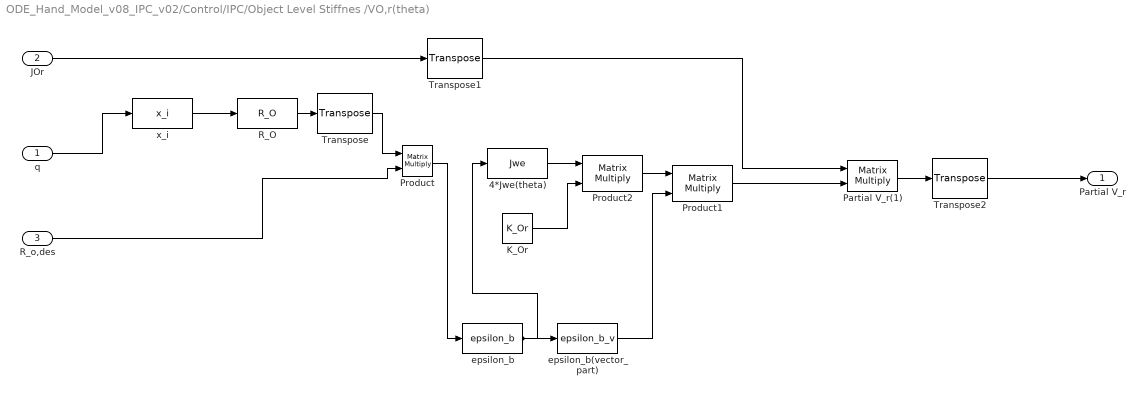
== system ODE_Hand_Model_v08_IPC_v02/Control/IPC/Object Level Stiffnes /VO,r(theta) ==
  q : Inport  OutDataType=fixdt(1, 16)  OutScaling=2^0
  JOr : Inport  Port=2  OutDataType=fixdt(1, 16)  OutScaling=2^0
  R_o,des : Inport  Port=3  OutDataType=fixdt(1, 16)  OutScaling=2^0
  4*Jwe(theta) : MATLABFcn  MATLABFcn=Jwe  Output1D=off
  K_Or : Constant  Value=K_Or  OutDataType=fixdt(1, 16)  OutScaling=2^0
  Partial V_r(1) : Product  Multiplication=Matrix(*)  OutDataType=fixdt(1, 16)  OutScaling=2^0  RndMeth=Zero
  Product : Product  Multiplication=Matrix(*)  OutDataType=fixdt(1, 16)  OutScaling=2^0  RndMeth=Zero
  Product1 : Product  Multiplication=Matrix(*)  OutDataType=fixdt(1, 16)  OutScaling=2^0  RndMeth=Zero
  Product2 : Product  Multiplication=Matrix(*)  OutDataType=fixdt(1, 16)  OutScaling=2^0  RndMeth=Zero
  R_O : MATLABFcn  MATLABFcn=R_O  OutputSignalType=real  Output1D=off
  Transpose : dspmtrx3/Transpose  SystemSampleTime=-1  Hermitian=off  overflowFlag=off
  Transpose1 : dspmtrx3/Transpose  SystemSampleTime=-1  Hermitian=off  overflowFlag=off
  Transpose2 : dspmtrx3/Transpose  SystemSampleTime=-1  Hermitian=off  overflowFlag=off
  epsilon_b : MATLABFcn  MATLABFcn=epsilon_b  Output1D=off
  epsilon_b(vector_part) : MATLABFcn  MATLABFcn=epsilon_b_v  Output1D=off
  x_i : MATLABFcn  MATLABFcn=x_i  Output1D=off
  Partial V_r : Outport  OutDataType=fixdt(1, 16)  OutScaling=2^0
  wires:
  q/1 -> x_i/1
  x_i/1 -> R_O/1
  Product/1 -> epsilon_b/1
  Product1/1 -> Partial V_r(1)/2
  K_Or/1 -> Product2/2
  Product2/1 -> Product1/1
  epsilon_b/1 -> 4*Jwe(theta)/1, epsilon_b(vector_part)/1
  epsilon_b(vector_part)/1 -> Product1/2
  Transpose1/1 -> Partial V_r(1)/1
  R_O/1 -> Transpose/1
  Transpose/1 -> Product/1
  JOr/1 -> Transpose1/1
  Partial V_r(1)/1 -> Transpose2/1
  Transpose2/1 -> Partial V_r/1
  4*Jwe(theta)/1 -> Product2/1
  R_o,des/1 -> Product/2

== system ODE_Hand_Model_v08_IPC_v02/Control/IPC/Object Level Stiffnes /VO,t(theta) ==
  q : Inport  OutDataType=fixdt(1, 16)  OutScaling=2^0
  JOt : Inport  Port=2  OutDataType=fixdt(1, 16)  OutScaling=2^0
  x_o,des : Inport  Port=3  OutDataType=fixdt(1, 16)  OutScaling=2^0
  K_Ot : Constant  Value=K_Ot  OutDataType=fixdt(1, 16)  OutScaling=2^0
  Product : Product  Multiplication=Matrix(*)  OutDataType=fixdt(1, 16)  OutScaling=2^0  RndMeth=Zero
  Product1 : Product  Multiplication=Matrix(*)  OutDataType=fixdt(1, 16)  OutScaling=2^0  RndMeth=Zero
  Product2 : Product  Multiplication=Matrix(*)  OutDataType=fixdt(1, 16)  OutScaling=2^0  RndMeth=Zero
  R_O : MATLABFcn  MATLABFcn=R_O  OutputSignalType=real  Output1D=off
  Sum : Sum  Inputs=|+-  OutDataType=fixdt(1, 16)  OutScaling=2^0
  Transpose : dspmtrx3/Transpose  SystemSampleTime=-1  Hermitian=off  overflowFlag=off
  Transpose1 : dspmtrx3/Transpose  SystemSampleTime=-1  Hermitian=off  overflowFlag=off
  Transpose2 : dspmtrx3/Transpose  SystemSampleTime=-1  Hermitian=off  overflowFlag=off
  X_O : MATLABFcn  MATLABFcn=x_O
  x_i : MATLABFcn  MATLABFcn=x_i  Output1D=off
  Out1 : Outport  OutDataType=fixdt(1, 16)  OutScaling=2^0
  wires:
  q/1 -> x_i/1
  JOt/1 -> Transpose/1
  x_i/1 -> R_O/1, X_O/1
  R_O/1 -> Transpose1/1
  X_O/1 -> Sum/1
  Sum/1 -> Product1/2
  Product1/1 -> Product/2
  K_Ot/1 -> Product/1
  Product/1 -> Product2/2
  Transpose/1 -> Product2/1
  Product2/1 -> Transpose2/1
  Transpose2/1 -> Out1/1
  x_o,des/1 -> Sum/2
  Transpose1/1 -> Product1/1

== system ODE_Hand_Model_v08_IPC_v02/Control/Initial_Posture/Ramp_Singals_qd/Ramp ==
  Demux : Demux  Tag=STV Demux  Outputs=1
  FromWs : FromWorkspace  Tag=STV FromWs  VariableName=tuvar  SampleTime=0  SigBuilderData=DataTag0  VnvData=DataTag1
      SigBuilderData=|
      | common.afterFinalStr = 'Extrapolate'
      | common.sampleTime = 0
      | dataSet.timeRange = [0 10]
      | dataSet.name = 'Group 1'
      | sbobj.Groups.Name = 'Group 1'
      | sbobj.Groups.Signals.Name = 'Signal 1'
      | sbobj.Groups.Signals.XData = [0 0.7 6 10]
      | sbobj.Groups.Signals.YData = [0 1 1 1]
  Signal 1 : Outport  Tag=STV Outport  OutDataType=fixdt(1, 16)  OutScaling=2^0
  wires:
  Demux/1 -> Signal 1/1
  FromWs/1 -> Demux/1

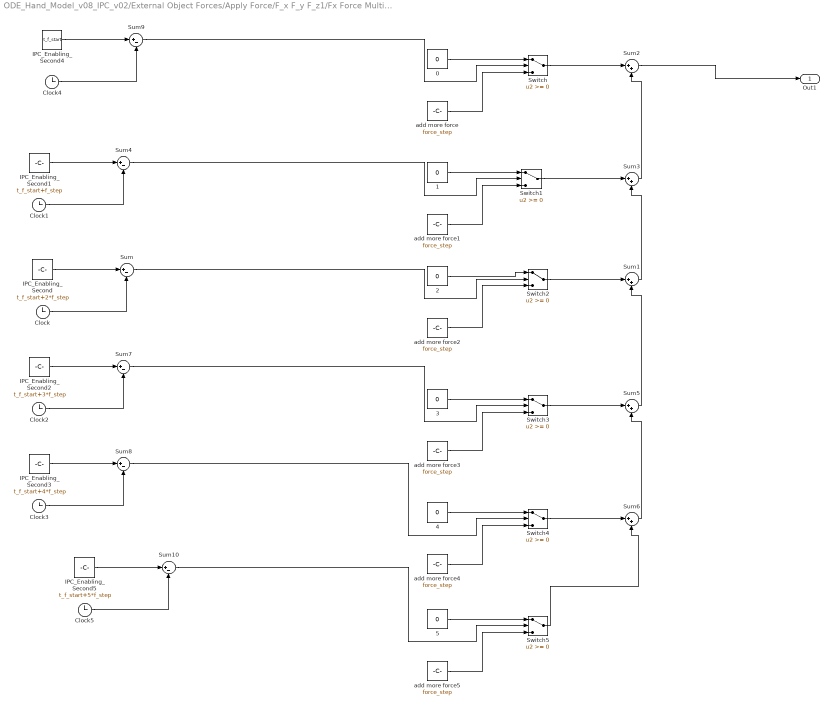
== system ODE_Hand_Model_v08_IPC_v02/External Object Forces/Apply Force/F_x F_y F_z1/Fx Force Multiplier ==
  {0..5} (6 alike) : Constant  Value=0  OutDataType=fixdt(1, 16)  OutScaling=2^0
  Clock{,1..5} (6 alike) : Clock
      settings: Decimation=10
  IPC_Enabling_Second : Constant  Value=t_f_start+2*f_step  OutDataType=fixdt(1, 16)  OutScaling=2^0
  IPC_Enabling_Second1 : Constant  Value=t_f_start+f_step  OutDataType=fixdt(1, 16)  OutScaling=2^0
  IPC_Enabling_Second2 : Constant  Value=t_f_start+3*f_step  OutDataType=fixdt(1, 16)  OutScaling=2^0
  IPC_Enabling_Second3 : Constant  Value=t_f_start+4*f_step  OutDataType=fixdt(1, 16)  OutScaling=2^0
  IPC_Enabling_Second4 : Constant  Value=t_f_start  OutDataType=fixdt(1, 16)  OutScaling=2^0
  IPC_Enabling_Second5 : Constant  Value=t_f_start+5*f_step  OutDataType=fixdt(1, 16)  OutScaling=2^0
  Sum{,4,7..10} (6 alike) : Sum  Inputs=|+-  OutDataType=fixdt(1, 16)  OutScaling=2^0
  Sum{1..3,5..6} (5 alike) : Sum  Inputs=|++  OutDataType=fixdt(1, 16)  OutScaling=2^0
  Switch{,1..5} (6 alike) : Switch  OutDataType=fixdt(1, 16)  OutScaling=2^0
  add more force{,1..5} (6 alike) : Constant  Value=force_step  OutDataType=fixdt(1, 16)  OutScaling=2^0
  Out1 : Outport  OutDataType=fixdt(1, 16)  OutScaling=2^0
  wires:
  0/1 -> Switch/1
  add more force/1 -> Switch/3
  Switch/1 -> Sum2/1
  1/1 -> Switch1/1
  add more force1/1 -> Switch1/3
  Switch1/1 -> Sum3/1
  2/1 -> Switch2/1
  add more force2/1 -> Switch2/3
  Switch2/1 -> Sum1/1
  add more force3/1 -> Switch3/3
  Switch3/1 -> Sum5/1
  4/1 -> Switch4/1
  add more force4/1 -> Switch4/3
  Switch4/1 -> Sum6/1
  5/1 -> Switch5/1
  add more force5/1 -> Switch5/3
  Switch5/1 -> Sum6/2
  Sum3/1 -> Sum2/2
  Sum1/1 -> Sum3/2
  Sum5/1 -> Sum1/2
  Sum6/1 -> Sum5/2
  Clock/1 -> Sum/2
  IPC_Enabling_Second/1 -> Sum/1
  Clock1/1 -> Sum4/2
  IPC_Enabling_Second1/1 -> Sum4/1
  Clock2/1 -> Sum7/2
  IPC_Enabling_Second2/1 -> Sum7/1
  Clock4/1 -> Sum9/2
  IPC_Enabling_Second4/1 -> Sum9/1
  Clock3/1 -> Sum8/2
  IPC_Enabling_Second3/1 -> Sum8/1
  Clock5/1 -> Sum10/2
  IPC_Enabling_Second5/1 -> Sum10/1
  Sum2/1 -> Out1/1
  Sum9/1 -> Switch/2
  Sum4/1 -> Switch1/2
  Sum/1 -> Switch2/2
  3/1 -> Switch3/1
  Sum7/1 -> Switch3/2
  Sum8/1 -> Switch4/2
  Sum10/1 -> Switch5/2

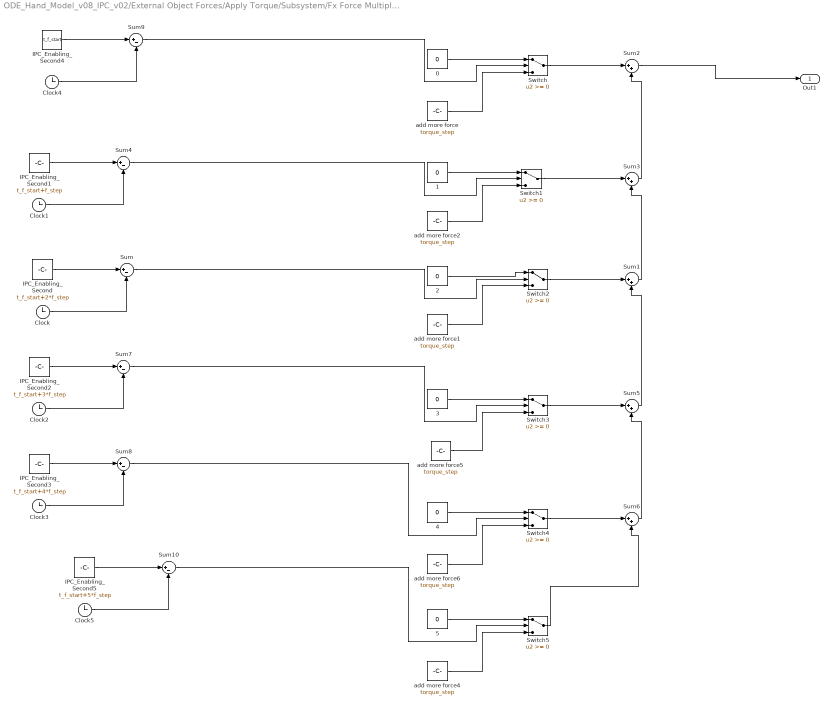
== system ODE_Hand_Model_v08_IPC_v02/External Object Forces/Apply Torque/Subsystem/Fx Force Multiplier ==
  {0..5} (6 alike) : Constant  Value=0  OutDataType=fixdt(1, 16)  OutScaling=2^0
  Clock{,1..5} (6 alike) : Clock
      settings: Decimation=10
  IPC_Enabling_Second : Constant  Value=t_f_start+2*f_step  OutDataType=fixdt(1, 16)  OutScaling=2^0
  IPC_Enabling_Second1 : Constant  Value=t_f_start+f_step  OutDataType=fixdt(1, 16)  OutScaling=2^0
  IPC_Enabling_Second2 : Constant  Value=t_f_start+3*f_step  OutDataType=fixdt(1, 16)  OutScaling=2^0
  IPC_Enabling_Second3 : Constant  Value=t_f_start+4*f_step  OutDataType=fixdt(1, 16)  OutScaling=2^0
  IPC_Enabling_Second4 : Constant  Value=t_f_start  OutDataType=fixdt(1, 16)  OutScaling=2^0
  IPC_Enabling_Second5 : Constant  Value=t_f_start+5*f_step  OutDataType=fixdt(1, 16)  OutScaling=2^0
  Sum{,4,7..10} (6 alike) : Sum  Inputs=|+-  OutDataType=fixdt(1, 16)  OutScaling=2^0
  Sum{1..3,5..6} (5 alike) : Sum  Inputs=|++  OutDataType=fixdt(1, 16)  OutScaling=2^0
  Switch{,1..5} (6 alike) : Switch  OutDataType=fixdt(1, 16)  OutScaling=2^0
  add more force{,1..2,4..6} (6 alike) : Constant  Value=torque_step  OutDataType=fixdt(1, 16)  OutScaling=2^0
  Out1 : Outport  OutDataType=fixdt(1, 16)  OutScaling=2^0
  wires:
  0/1 -> Switch/1
  add more force/1 -> Switch/3
  Switch/1 -> Sum2/1
  1/1 -> Switch1/1
  add more force2/1 -> Switch1/3
  Switch1/1 -> Sum3/1
  2/1 -> Switch2/1
  add more force1/1 -> Switch2/3
  Switch2/1 -> Sum1/1
  add more force5/1 -> Switch3/3
  Switch3/1 -> Sum5/1
  4/1 -> Switch4/1
  add more force6/1 -> Switch4/3
  Switch4/1 -> Sum6/1
  5/1 -> Switch5/1
  add more force4/1 -> Switch5/3
  Switch5/1 -> Sum6/2
  Sum3/1 -> Sum2/2
  Sum1/1 -> Sum3/2
  Sum5/1 -> Sum1/2
  Sum6/1 -> Sum5/2
  Clock/1 -> Sum/2
  IPC_Enabling_Second/1 -> Sum/1
  Clock1/1 -> Sum4/2
  IPC_Enabling_Second1/1 -> Sum4/1
  Clock2/1 -> Sum7/2
  IPC_Enabling_Second2/1 -> Sum7/1
  Clock4/1 -> Sum9/2
  IPC_Enabling_Second4/1 -> Sum9/1
  Clock3/1 -> Sum8/2
  IPC_Enabling_Second3/1 -> Sum8/1
  Clock5/1 -> Sum10/2
  IPC_Enabling_Second5/1 -> Sum10/1
  Sum2/1 -> Out1/1
  Sum9/1 -> Switch/2
  Sum4/1 -> Switch1/2
  Sum/1 -> Switch2/2
  3/1 -> Switch3/1
  Sum7/1 -> Switch3/2
  Sum8/1 -> Switch4/2
  Sum10/1 -> Switch5/2

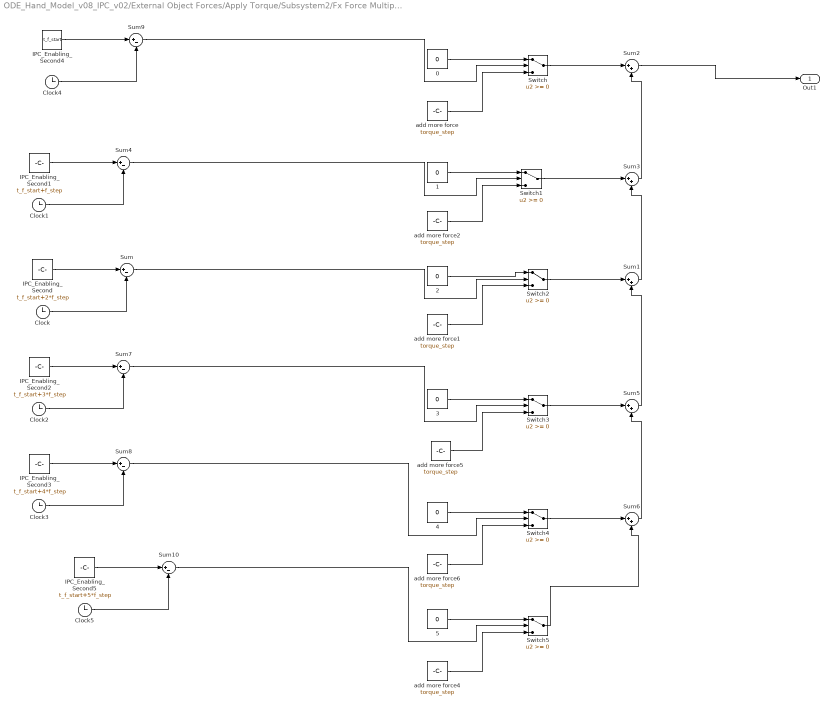
== system ODE_Hand_Model_v08_IPC_v02/External Object Forces/Apply Torque/Subsystem2/Fx Force Multiplier ==
  {0..5} (6 alike) : Constant  Value=0  OutDataType=fixdt(1, 16)  OutScaling=2^0
  Clock{,1..5} (6 alike) : Clock
      settings: Decimation=10
  IPC_Enabling_Second : Constant  Value=t_f_start+2*f_step  OutDataType=fixdt(1, 16)  OutScaling=2^0
  IPC_Enabling_Second1 : Constant  Value=t_f_start+f_step  OutDataType=fixdt(1, 16)  OutScaling=2^0
  IPC_Enabling_Second2 : Constant  Value=t_f_start+3*f_step  OutDataType=fixdt(1, 16)  OutScaling=2^0
  IPC_Enabling_Second3 : Constant  Value=t_f_start+4*f_step  OutDataType=fixdt(1, 16)  OutScaling=2^0
  IPC_Enabling_Second4 : Constant  Value=t_f_start  OutDataType=fixdt(1, 16)  OutScaling=2^0
  IPC_Enabling_Second5 : Constant  Value=t_f_start+5*f_step  OutDataType=fixdt(1, 16)  OutScaling=2^0
  Sum{,4,7..10} (6 alike) : Sum  Inputs=|+-  OutDataType=fixdt(1, 16)  OutScaling=2^0
  Sum{1..3,5..6} (5 alike) : Sum  Inputs=|++  OutDataType=fixdt(1, 16)  OutScaling=2^0
  Switch{,1..5} (6 alike) : Switch  OutDataType=fixdt(1, 16)  OutScaling=2^0
  add more force{,1..2,4..6} (6 alike) : Constant  Value=torque_step  OutDataType=fixdt(1, 16)  OutScaling=2^0
  Out1 : Outport  OutDataType=fixdt(1, 16)  OutScaling=2^0
  wires:
  0/1 -> Switch/1
  add more force/1 -> Switch/3
  Switch/1 -> Sum2/1
  1/1 -> Switch1/1
  add more force2/1 -> Switch1/3
  Switch1/1 -> Sum3/1
  2/1 -> Switch2/1
  add more force1/1 -> Switch2/3
  Switch2/1 -> Sum1/1
  add more force5/1 -> Switch3/3
  Switch3/1 -> Sum5/1
  4/1 -> Switch4/1
  add more force6/1 -> Switch4/3
  Switch4/1 -> Sum6/1
  5/1 -> Switch5/1
  add more force4/1 -> Switch5/3
  Switch5/1 -> Sum6/2
  Sum3/1 -> Sum2/2
  Sum1/1 -> Sum3/2
  Sum5/1 -> Sum1/2
  Sum6/1 -> Sum5/2
  Clock/1 -> Sum/2
  IPC_Enabling_Second/1 -> Sum/1
  Clock1/1 -> Sum4/2
  IPC_Enabling_Second1/1 -> Sum4/1
  Clock2/1 -> Sum7/2
  IPC_Enabling_Second2/1 -> Sum7/1
  Clock4/1 -> Sum9/2
  IPC_Enabling_Second4/1 -> Sum9/1
  Clock3/1 -> Sum8/2
  IPC_Enabling_Second3/1 -> Sum8/1
  Clock5/1 -> Sum10/2
  IPC_Enabling_Second5/1 -> Sum10/1
  Sum2/1 -> Out1/1
  Sum9/1 -> Switch/2
  Sum4/1 -> Switch1/2
  Sum/1 -> Switch2/2
  3/1 -> Switch3/1
  Sum7/1 -> Switch3/2
  Sum8/1 -> Switch4/2
  Sum10/1 -> Switch5/2
